simulink model "CP_model"  (R2015a)
settings: Solver=ode45  StartTime=0.0  StopTime=6  RelTol=1e-3
libraries: fuzblock x1, simulink x1
settings Model: Creator=root  LastModifiedBy=rojas-j

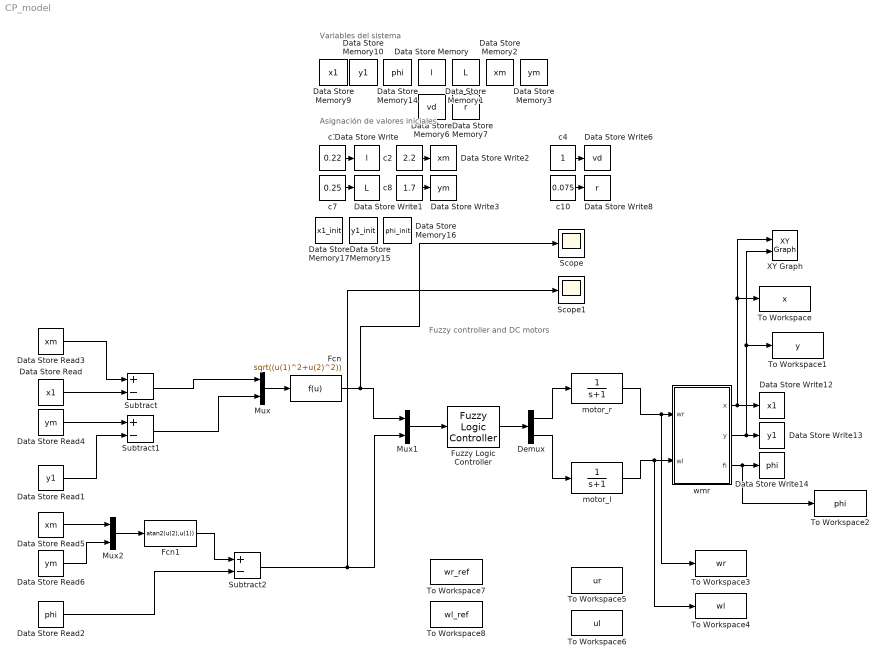
== system CP_model ==
  note: Fuzzy controller and DC motors
  note: Variables del sistema
  note: Asignación de valores iniciales
  Data Store Memory : DataStoreMemory  DataStoreName=l  ReadBeforeWriteMsg=warning  WriteAfterWriteMsg=warning  WriteAfterReadMsg=warning
  Data Store Memory1 : DataStoreMemory  DataStoreName=L  ReadBeforeWriteMsg=warning  WriteAfterWriteMsg=warning  WriteAfterReadMsg=warning
  Data Store Memory10 : DataStoreMemory  DataStoreName=y1  ReadBeforeWriteMsg=warning  WriteAfterWriteMsg=warning  WriteAfterReadMsg=warning
  Data Store Memory14 : DataStoreMemory  DataStoreName=phi  ReadBeforeWriteMsg=warning  WriteAfterWriteMsg=warning  WriteAfterReadMsg=warning
  Data Store Memory15 : DataStoreMemory  DataStoreName=y1_init  ReadBeforeWriteMsg=warning  WriteAfterWriteMsg=warning  WriteAfterReadMsg=warning
  Data Store Memory16 : DataStoreMemory  DataStoreName=phi_init  ReadBeforeWriteMsg=warning  WriteAfterWriteMsg=warning  WriteAfterReadMsg=warning
  Data Store Memory17 : DataStoreMemory  DataStoreName=x1_init  ReadBeforeWriteMsg=warning  WriteAfterWriteMsg=warning  WriteAfterReadMsg=warning
  Data Store Memory2 : DataStoreMemory  DataStoreName=xm  ReadBeforeWriteMsg=warning  WriteAfterWriteMsg=warning  WriteAfterReadMsg=warning
  Data Store Memory3 : DataStoreMemory  DataStoreName=ym  ReadBeforeWriteMsg=warning  WriteAfterWriteMsg=warning  WriteAfterReadMsg=warning
  Data Store Memory6 : DataStoreMemory  DataStoreName=vd  ReadBeforeWriteMsg=warning  WriteAfterWriteMsg=warning  WriteAfterReadMsg=warning
  Data Store Memory7 : DataStoreMemory  DataStoreName=r  ReadBeforeWriteMsg=warning  WriteAfterWriteMsg=warning  WriteAfterReadMsg=warning
  Data Store Memory9 : DataStoreMemory  DataStoreName=x1  ReadBeforeWriteMsg=warning  WriteAfterWriteMsg=warning  WriteAfterReadMsg=warning
  Data Store Read : DataStoreRead  DataStoreName=x1
  Data Store Read1 : DataStoreRead  DataStoreName=y1
  Data Store Read2 : DataStoreRead  DataStoreName=phi
  Data Store Read3 : DataStoreRead  DataStoreName=xm
  Data Store Read4 : DataStoreRead  DataStoreName=ym
  Data Store Read5 : DataStoreRead  DataStoreName=xm
  Data Store Read6 : DataStoreRead  DataStoreName=ym
  Data Store Write : DataStoreWrite  DataStoreName=l
  Data Store Write1 : DataStoreWrite  DataStoreName=L
  Data Store Write12 : DataStoreWrite  DataStoreName=x1
  Data Store Write13 : DataStoreWrite  DataStoreName=y1
  Data Store Write14 : DataStoreWrite  DataStoreName=phi
  Data Store Write2 : DataStoreWrite  DataStoreName=xm
  Data Store Write3 : DataStoreWrite  DataStoreName=ym
  Data Store Write6 : DataStoreWrite  DataStoreName=vd
  Data Store Write8 : DataStoreWrite  DataStoreName=r
  Demux : Demux  Outputs=2
  Fcn : Fcn  Expr=sqrt((u(1)^2+u(2)^2))
  Fcn1 : Fcn  Expr=atan2(u(2),u(1))
  Fuzzy Logic Controller : fuzblock/Fuzzy Logic  Controller  fis='caldera.fis'
  Mux : Mux  Inputs=2
  Mux1 : Mux  Inputs=2
  Mux2 : Mux  Inputs=2
  Scope : Scope
  Scope1 : Scope
  Subtract : Sum  Inputs=+-
  Subtract1 : Sum  Inputs=+-
  Subtract2 : Sum  Inputs=+-
  To Workspace : ToWorkspace  VariableName=x  SaveFormat=Timeseries  SampleTime=-1
  To Workspace1 : ToWorkspace  VariableName=y  SaveFormat=Timeseries  SampleTime=-1
  To Workspace2 : ToWorkspace  VariableName=phi  SaveFormat=Timeseries  SampleTime=-1
  To Workspace3 : ToWorkspace  VariableName=wr  SaveFormat=Timeseries  SampleTime=-1
  To Workspace4 : ToWorkspace  VariableName=wl  SaveFormat=Timeseries  SampleTime=-1
  To Workspace5 : ToWorkspace  VariableName=ur  SaveFormat=Timeseries  SampleTime=-1
  To Workspace6 : ToWorkspace  VariableName=ul  SaveFormat=Timeseries  SampleTime=-1
  To Workspace7 : ToWorkspace  VariableName=wr_ref  SaveFormat=Timeseries  SampleTime=-1
  To Workspace8 : ToWorkspace  VariableName=wl_ref  SaveFormat=Timeseries  SampleTime=-1
  XY Graph : simulink/Sinks/XY Graph  xmin=-1  xmax=1  ymin=-1  ymax=1  st=-1
  "c1 " : Constant  Value=0.22
  c10 : Constant  Value=0.075
  c2 : Constant  Value=2.2
  c4 : Constant
  c7 : Constant  Value=0.25
  c8 : Constant  Value=1.7
  motor_l : TransferFcn  Denominator=[1 1]
  motor_r : TransferFcn  Denominator=[1 1]
  wmr : Subsystem
  wires:
  "c1 "/1 -> Data Store Write/1
  c7/1 -> Data Store Write1/1
  c2/1 -> Data Store Write2/1
  c8/1 -> Data Store Write3/1
  c4/1 -> Data Store Write6/1
  c10/1 -> Data Store Write8/1
  Data Store Read/1 -> Subtract/2
  motor_l/1 -> To Workspace4/1, wmr/2(wl)
  wmr/2(y) -> XY Graph/2, To Workspace1/1, Data Store Write13/1
  wmr/1(x) -> XY Graph/1, To Workspace/1, Data Store Write12/1
  wmr/3(fi) -> To Workspace2/1, Data Store Write14/1
  motor_r/1 -> To Workspace3/1, wmr/1(wr)
  Data Store Read3/1 -> Subtract/1
  Data Store Read1/1 -> Subtract1/2
  Data Store Read4/1 -> Subtract1/1
  Fuzzy Logic Controller/1 -> Demux/1
  Data Store Read2/1 -> Subtract2/2
  Demux/1 -> motor_r/1
  Demux/2 -> motor_l/1
  Subtract/1 -> Mux/1
  Subtract1/1 -> Mux/2
  Mux/1 -> Fcn/1
  Fcn/1 -> Scope/1, Mux1/1
  Data Store Read5/1 -> Mux2/1
  Data Store Read6/1 -> Mux2/2
  Mux2/1 -> Fcn1/1
  Fcn1/1 -> Subtract2/1
  Subtract2/1 -> Scope1/1, Mux1/2
  Mux1/1 -> Fuzzy Logic Controller/1

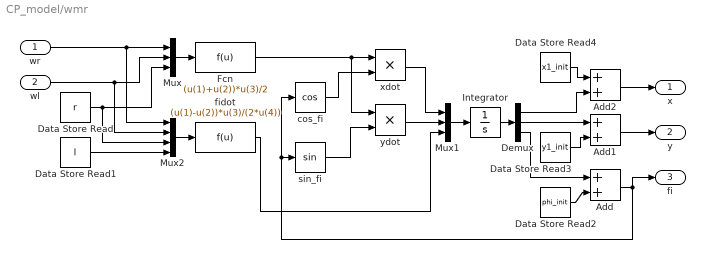
== system CP_model/wmr ==
  wr : Inport
  wl : Inport  Port=2
  Add : Sum
  Add1 : Sum
  Add2 : Sum
  Data Store Read : DataStoreRead  DataStoreName=r
  Data Store Read1 : DataStoreRead  DataStoreName=l
  Data Store Read2 : DataStoreRead  DataStoreName=phi_init
  Data Store Read3 : DataStoreRead  DataStoreName=y1_init
  Data Store Read4 : DataStoreRead  DataStoreName=x1_init
  Demux : Demux  Outputs=3
  Fcn : Fcn  Expr=(u(1)+u(2))*u(3)/2
  Integrator : Integrator
  Mux : Mux  Inputs=3
  Mux1 : Mux  Inputs=3
  Mux2 : Mux
  "cos_fi " : Trigonometry  Operator=cos
  fidot : Fcn  Expr=(u(1)-u(2))*u(3)/(2*u(4))
  "sin_fi " : Trigonometry
  xdot : Product
  ydot : Product
  x : Outport
  y : Outport  Port=2
  fi : Outport  Port=3
  wires:
  wr/1 -> Mux2/1, Mux/1
  wl/1 -> Mux2/2, Mux/2
  Mux/1 -> Fcn/1
  Mux1/1 -> Integrator/1
  Integrator/1 -> Demux/1
  Fcn/1 -> xdot/1, ydot/1
  "cos_fi "/1 -> xdot/2
  xdot/1 -> Mux1/1
  "sin_fi "/1 -> ydot/2
  Data Store Read/1 -> Mux2/3, Mux/3
  ydot/1 -> Mux1/2
  Mux2/1 -> fidot/1
  fidot/1 -> Mux1/3
  Data Store Read1/1 -> Mux2/4
  Demux/3 -> Add/1
  Data Store Read2/1 -> Add/2
  Add/1 -> fi/1, "cos_fi "/1, "sin_fi "/1
  Add1/1 -> y/1
  Data Store Read3/1 -> Add1/2
  Demux/2 -> Add1/1
  Demux/1 -> Add2/2
  Data Store Read4/1 -> Add2/1
  Add2/1 -> x/1
